simulink model "DYC_controller"  (R2018b)
settings: Solver=FixedStepAuto  StartTime=0.0  StopTime=inf  FixedStep=Ts  RelTol=1e-3  EnableMultiTasking=on
values from neighbouring files (symbols this model uses):
  A_vte = [1 0 -2*Ts*m_s/WB*(l_r*h_rc_f/w1+l_f*h_rc_r/w2) 0 -2*Ts*(K_f/w1+K_r/w2) ... (first row only)    [main.m]
  A_vte_p2 = [1 0 0 0 0 -Ts * m * hc / 2 / WB 0 -Ts * l_r * m * hc / WB / w1 ... (first row only)    [main.m]
  b1 = ones(4,1)/R    [main.m]
  boundary = 3000    [main.m]
  C_vte = [0 1 0 g 0 ... (first row only)    [main.m]
  C_vte_p2 = [1, -1, 1, -1, 0, 0, 0, 0 ... (first row only)    [main.m]
  eta = 0    [main.m]
  F_z1_s = l_r * m * g / 2 / WB    (= 9.45353456158)    [main.m]
  F_z2_s = F_z1_s    (= 9.45353456158)    [main.m]
  F_z3_s = l_f * m * g / 2 / WB    (= 9.11094809852)    [main.m]
  F_z4_s = F_z3_s    (= 9.11094809852)    [main.m]
  g = 9.81    [main.m]
  h_rc_f = 0.00    (= 0)    [main.m]
  h_rc_r = 0.00    (= 0)    [main.m]
  hc = 0.0751    [main.m]
  J = 0.9    [main.m]
  k1 = 2000    [main.m]
  k2 = 1000    [main.m]
  K_f = K_lin*l_cs^2*cos(phi*pi/180)    [main.m]
  K_r = K_lin*l_cs^2*cos(phi*pi/180)    [main.m]
  Kd = 0    [main.m]
  Ki = 75    [main.m]
  Kp = 600    [main.m]
  l_f = 0.1968    [main.m]
  l_r = 0.2042    [main.m]
  m = 3.832    [main.m]
  m_s = 0.9*m    (= 3.4488)    [main.m]
  mu = 0.8    [main.m]
  Protean_PD18_motormap = [2.92104016907 601.978033502 650.789692516 685.109940533 725.756581133 754.659963437 780.850883334 807.9513301 837.761936672 868.484372712 893.788791739 922.70944354 ... (50 elements, 25x2)]    [Protean_PD18_motormap.mat]
  Q_lat_process = 1E0*[var_r^2  0 0 0 0 0 0 0 0 ... (first row only)    [main.m]
  Q_lat_sensor = 1E-2*[var_r_s^2 0 0 0 ... (first row only)    [main.m]
  Q_meas_susp_p1 = [var_ay_m_p^2 0 0 0 ... (first row only)    [main.m]
  Q_meas_susp_p2 = [var_del_Fz^2 0 0 0 0 ... (first row only)    [main.m]
  R = 0.055    [main.m]
  Ts = 0.015    [main.m]
  V_x0 = (1000/3600)*V_x0    (= 11.1111111111)    [main.m]
  w1 = 0.2824    [main.m]
  w2 = 2.929    [main.m]
  WB = 0.406    [main.m]
undefined symbols (not defined in the file or in its folder): C_lf, C_lr, DiscIntNeverNeededParam, Discrete, t_e, Time
libraries: raspberrypilib x24, hdlsllib x21, simulink x17, discretizing x2, ctrlSharedLib x2, sharedTrackingLibrary x1
(part 1 of 3)
settings Model: SimulationMode=external  Creator=domin  LastModifiedBy=Heisenberg
settings SolverCC: ConcurrentTasks=on  PositivePriorityOrder=on  AutoInsertRateTranBlk=on
settings DataIOCC: SaveFormat=Array
settings OptimizationCC: EnhancedBackFolding=on  PassReuseOutputArgsThreshold=0  MaxStackSize=64  OptimizeBlockOrder=speed  DifferentSizesBufferReuse=on  OptimizationCustomize=off
settings DebuggingCC: ParameterTunabilityLossMsg=error  LibraryContextMissingDiagnostic=none
settings HardwareCC: ProdBitPerPointer=32  ProdBitPerSizeT=32  ProdBitPerPtrDiffT=32  ProdLargestAtomicInteger=Long  ProdLargestAtomicFloat=Double  ProdWordSize=32  ProdHWDeviceType=ARM Compatible->ARM Cortex  UseEmbeddedCoderFeatures=off  UseSimulinkCoderFeatures=off
settings ModelReferenceCC: ModelReferenceMinAlgLoopOccurrences=on
settings SFSimCC: SimUseLocalCustomCode=off  MATLABDynamicMemAlloc=off
settings RTWCC: SystemTargetFile=ert.tlc  HardwareBoard=Raspberry Pi  TLCOptions="-aInlineSetEventsForThisBaseRateFcn=TLC_FALSE -aSuppressMultiTaskScheduler=TLC_FALSE  -aRateBasedStepFcn=0"  TemplateMakefile=ert_default_tmf  RTWVerbose=off  RTWUseLocalCustomCode=off  Toolchain=GNU GCC Raspberry Pi  BuildConfiguration=Faster Runs
settings CodeAppCC: ForceParamTrailComments=on  OperatorAnnotations=on  MangleLength=10
settings ERTTargetCC: ERTCustomFileBanners=off  SupportContinuousTime=on  SupportNonInlinedSFcns=on  RemoveResetFunc=off  SupportVariableSizeSignals=on  ModelStepFunctionPrototypeControlCompliant=off  ExtMode=on  ExtModeMexArgs='192.168.1.5' 0 17725  ERTSrcFileBannerTemplate=codertarget_code_template.cgt  ERTHdrFileBannerTemplate=codertarget_code_template.cgt  ERTDataSrcFileTemplate=codertarget_code_template.cgt  ERTDataHdrFileTemplate=codertarget_code_template.cgt

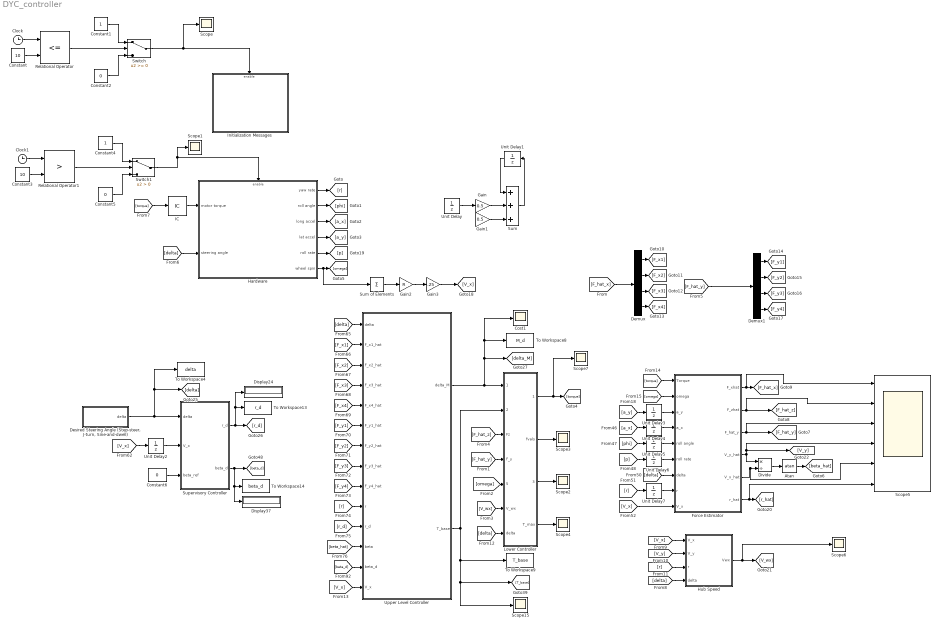
== system DYC_controller ==
  Atan : Trigonometry  Operator=atan
  Clock : Clock
  Clock1 : Clock
  Constant : Constant  Value=10
  Constant1 : Constant
  Constant2 : Constant  Value=0
  Constant3 : Constant  Value=10
  Constant4 : Constant
  Constant5 : Constant  Value=0
  Constant6 : Constant  Value=0  SampleTime=Ts
  Cost1 : Scope
  Demux : Demux
  Demux1 : Demux
  "Desired Steering Angle (Step-steer, J-turn, Sine-and-dwell)" : Subsystem
  Display24 : Display
  Display37 : Display
  Divide : Product  Inputs=*/
  Force Estimator : Subsystem
  Gain : Gain  Gain=0.5
  Gain1 : Gain  Gain=0.5
  Gain2 : Gain  Gain=R
  Gain3 : Gain  Gain=.25
  Hardware : Subsystem
  Hub Speed : Subsystem
  IC : InitialCondition  Value=0
  Initialization Messages : Subsystem
  Lower Controller : Subsystem
  Relational Operator : RelationalOperator  Operator=<=  OutDataTypeStr=boolean  RndMeth=Simplest
  Relational Operator1 : RelationalOperator  Operator=>  OutDataTypeStr=boolean  RndMeth=Simplest
  Scope{,1..4,6..7,15} (8 alike) : Scope
  Scope5 : Scope  NumInputPorts=6
  Sum : Sum  Inputs=+++
  Sum of Elements : Sum  Inputs=+
  "Supervisory Controller " : Subsystem
  Switch : Switch
  Switch1 : Switch  Criteria=u2 > Threshold
  To Workspace13 : ToWorkspace  VariableName=r_d  SampleTime=-1
  To Workspace14 : ToWorkspace  VariableName=beta_d  SampleTime=-1
  To Workspace4 : ToWorkspace  VariableName=delta  SampleTime=-1
  To Workspace8 : ToWorkspace  VariableName=M_d  SampleTime=-1
  To Workspace9 : ToWorkspace  VariableName=T_base  SampleTime=-1
  Unit Delay{,1..7} (8 alike) : UnitDelay  SampleTime=-1
  Upper Level Controller : Subsystem
  wires:
  Clock/1 -> Relational Operator/1
  Constant/1 -> Relational Operator/2
  Relational Operator/1 -> Switch/2
  Constant1/1 -> Switch/1
  Constant2/1 -> Switch/3
  Switch/1 -> Scope/1, Initialization Messages/Enable
  Switch1/1 -> Scope1/1, Hardware/Enable
  Constant5/1 -> Switch1/3
  Constant4/1 -> Switch1/1
  Relational Operator1/1 -> Switch1/2
  Constant3/1 -> Relational Operator1/2
  Clock1/1 -> Relational Operator1/1
  "Supervisory Controller "/1(r_d) -> Display24/1, To Workspace13/1, [r_d]
  Constant6/1 -> "Supervisory Controller "/3(beta_ref)
  [V_x] -> Unit Delay2/1
  "Desired Steering Angle (Step-steer, J-turn, Sine-and-dwell)"/1(delta) -> To Workspace4/1, [delta], "Supervisory Controller "/1(delta)
  "Supervisory Controller "/2(beta_d) -> To Workspace14/1, Display37/1, [beta_d]
  [F_x1] -> Upper Level Controller/2(F_x1_hat)
  [delta] -> Lower Controller/7(delta)
  [F_y3] -> Upper Level Controller/8(F_y3_hat)
  Upper Level Controller/1(delta_M) -> Cost1/1, To Workspace8/1, [delta_M], Lower Controller/1(delta_M)
  [F_x3] -> Upper Level Controller/4(F_x3_hat)
  [F_y1] -> Upper Level Controller/6(F_y1_hat)
  [F_y4] -> Upper Level Controller/9(F_y4_hat)
  Upper Level Controller/2(T_base) -> To Workspace9/1, [T_base], Scope15/1, Lower Controller/2(T_base)
  [F_hat_y] -> Lower Controller/4(F_y)
  [r_d] -> Upper Level Controller/11(r_d)
  [F_x4] -> Upper Level Controller/5(F_x4_hat)
  [V_wx] -> Lower Controller/6(V_wx)
  [r] -> Upper Level Controller/10(r)
  [V_x] -> Upper Level Controller/14(V_x)
  [delta] -> Upper Level Controller/1(delta)
  [beta_d] -> Upper Level Controller/13(beta_d)
  [F_hat_z] -> Lower Controller/3(Fz)
  [F_x2] -> Upper Level Controller/3(F_x2_hat)
  [omega] -> Lower Controller/5(omega)
  [F_y2] -> Upper Level Controller/7(F_y2_hat)
  [beta_hat] -> Upper Level Controller/12(beta)
  [torque] -> Force Estimator/1(Torque)
  [a_y] -> Unit Delay3/1
  [p] -> Unit Delay6/1
  [delta] -> Force Estimator/7(delta)
  [a_x] -> Unit Delay4/1
  [r] -> Unit Delay7/1
  [phi] -> Unit Delay5/1
  [omega] -> Force Estimator/2(omega)
  Hardware/1(yaw rate) -> [r]
  Hardware/2(roll angle) -> [phi]
  Hardware/3(long accel) -> [a_x]
  Hardware/4(lat accel) -> [a_y]
  Hardware/6(wheel spin) -> Sum of Elements/1, [omega]
  Divide/1 -> Atan/1
  Force Estimator/4(V_y_hat) -> Scope5/4, [V_y], Divide/1
  Force Estimator/5(V_x_hat) -> Scope5/5, Divide/2
  Atan/1 -> [beta_hat]
  Force Estimator/3(F_hat_y) -> Scope5/3, [F_hat_y]
  Force Estimator/2(F_zhat) -> Scope5/2, [F_hat_z]
  Force Estimator/1(F_xhat) -> Scope5/1, [F_hat_x]
  [F_hat_x] -> Demux/1
  Demux/1 -> [F_x1]
  Demux/2 -> [F_x2]
  Demux/3 -> [F_x3]
  Demux/4 -> [F_x4]
  Demux1/4 -> [F_y4]
  Demux1/3 -> [F_y3]
  Demux1/2 -> [F_y2]
  Demux1/1 -> [F_y1]
  Unit Delay/1 -> Gain/1
  Gain/1 -> Sum/2
  Gain1/1 -> Sum/3
  Hardware/5(roll rate) -> [p]
  [delta] -> Hardware/2(steering angle)
  Force Estimator/6(r_hat) -> Scope5/6, [r_hat]
  Lower Controller/3(iterations) -> Scope2/1
  Lower Controller/2(fvals) -> Scope3/1
  Lower Controller/4(T_max) -> Scope4/1
  [delta] -> Hub Speed/4(delta)
  [V_y] -> Hub Speed/2(V_y)
  [r] -> Hub Speed/3(r)
  [V_x] -> Hub Speed/1("V_x ")
  Hub Speed/1(Vwx) -> Scope6/1, [V_wx]
  Lower Controller/1(Motor Torques) -> Scope7/1, [torque]
  [torque] -> IC/1
  [F_hat_y] -> Demux1/1
  Unit Delay1/1 -> Sum/1
  Unit Delay2/1 -> "Supervisory Controller "/2(V_x)
  IC/1 -> Hardware/1(motor torque)
  Unit Delay3/1 -> Force Estimator/3(a_y)
  Unit Delay4/1 -> Force Estimator/4(a_x)
  Unit Delay5/1 -> Force Estimator/5(roll angle)
  Unit Delay6/1 -> Force Estimator/6(roll rate)
  Unit Delay7/1 -> Force Estimator/8(r)
  [V_x] -> Force Estimator/9(V_x)
  Sum/1 -> Unit Delay1/1
  Sum of Elements/1 -> Gain2/1
  Gain2/1 -> Gain3/1
  Gain3/1 -> [V_x]

== system DYC_controller/Desired Steering Angle (Step-steer, J-turn, Sine-and-dwell) ==
  J-Turn : Subsystem
  delta : Outport
  wires:
  J-Turn/1(delta) -> delta/1

== system DYC_controller/Force Estimator ==
  Torque : Inport
  omega : Inport  Port=2
  a_y : Inport  Port=3
  a_x : Inport  Port=4
  roll angle : Inport  Port=5
  roll rate : Inport  Port=6
  delta : Inport  Port=7
  r : Inport  Port=8
  V_x : Inport  Port=9
  Gain : Gain  Gain=pi/180
  Gain1 : Gain  Gain=pi/180
  Gain2 : Gain  Gain=pi/180
  Lateral Tire Force Estimation : Subsystem
  Longitudinal Tire Force Estimation : Subsystem
  Mux : Mux
  Vertical Tire Force Estimation : Subsystem
  F_xhat : Outport
  F_zhat : Outport  Port=2
  F_hat_y : Outport  Port=3
  V_y_hat : Outport  Port=4
  V_x_hat : Outport  Port=5
  r_hat : Outport  Port=6
  wires:
  Torque/1 -> Longitudinal Tire Force Estimation/1(torque)
  Longitudinal Tire Force Estimation/1(F_hat_x1) -> Mux/1
  Longitudinal Tire Force Estimation/2(F_hat_x2) -> Mux/2
  Longitudinal Tire Force Estimation/3(F_hat_x3) -> Mux/3
  Longitudinal Tire Force Estimation/4(F_hat_x4) -> Mux/4
  Mux/1 -> F_xhat/1
  omega/1 -> Longitudinal Tire Force Estimation/2(omega)
  a_y/1 -> Vertical Tire Force Estimation/4(a_y)
  a_x/1 -> Vertical Tire Force Estimation/1(a_x)
  roll angle/1 -> Gain/1
  roll rate/1 -> Gain1/1
  delta/1 -> Lateral Tire Force Estimation/2(delta)
  r/1 -> Gain2/1
  V_x/1 -> Lateral Tire Force Estimation/4(V_x)
  Lateral Tire Force Estimation/1(r_hat) -> r_hat/1
  Vertical Tire Force Estimation/2(a_x_hat) -> Lateral Tire Force Estimation/5(a_x)
  Vertical Tire Force Estimation/3(a_y_hat) -> Lateral Tire Force Estimation/6(a_y)
  Vertical Tire Force Estimation/1(F_zhat) -> F_zhat/1, Lateral Tire Force Estimation/1(F_zhat)
  Lateral Tire Force Estimation/4(F_hat_y) -> F_hat_y/1
  Lateral Tire Force Estimation/3(V_y_hat) -> V_y_hat/1
  Lateral Tire Force Estimation/2(V_x_hat) -> V_x_hat/1
  Gain/1 -> Vertical Tire Force Estimation/2(roll angle)
  Gain1/1 -> Vertical Tire Force Estimation/3(roll rate)
  Gain2/1 -> Lateral Tire Force Estimation/3(r)

== system DYC_controller/Hardware ==
  motor torque : Inport
  steering angle : Inport  Port=2
  Enable : EnablePort
  Const Mot Vel : Constant  Value=50
  SSIV Hardware Communication : Subsystem
  Throttle and Steering Handler : Subsystem
  yaw rate : Outport
  roll angle : Outport  Port=2
  long accel : Outport  Port=3
  lat accel : Outport  Port=4
  roll rate : Outport  Port=5
  wheel spin : Outport  Port=6
  wires:
  Throttle and Steering Handler/1(Throttle RF) -> SSIV Hardware Communication/1(throttle_right_front)
  Throttle and Steering Handler/2(Throttle LF) -> SSIV Hardware Communication/2(throttle_left_front)
  Throttle and Steering Handler/3(Throttle RR) -> SSIV Hardware Communication/3(throttle_right_rear)
  Throttle and Steering Handler/4(Throttle LR) -> SSIV Hardware Communication/4(throttle_left_rear)
  Throttle and Steering Handler/5(Outport) -> SSIV Hardware Communication/5(servo_out)
  Const Mot Vel/1 -> Throttle and Steering Handler/2(Inport2)
  SSIV Hardware Communication/9(gyr_z) -> yaw rate/1
  SSIV Hardware Communication/3(euler_roll) -> roll angle/1
  SSIV Hardware Communication/4(acc_x) -> long accel/1
  SSIV Hardware Communication/6(acc_y) -> lat accel/1
  motor torque/1 -> Throttle and Steering Handler/1(throttle)
  steering angle/1 -> Throttle and Steering Handler/3(steering angle)
  SSIV Hardware Communication/7(gyr_y) -> roll rate/1
  SSIV Hardware Communication/12(wheel spin) -> wheel spin/1

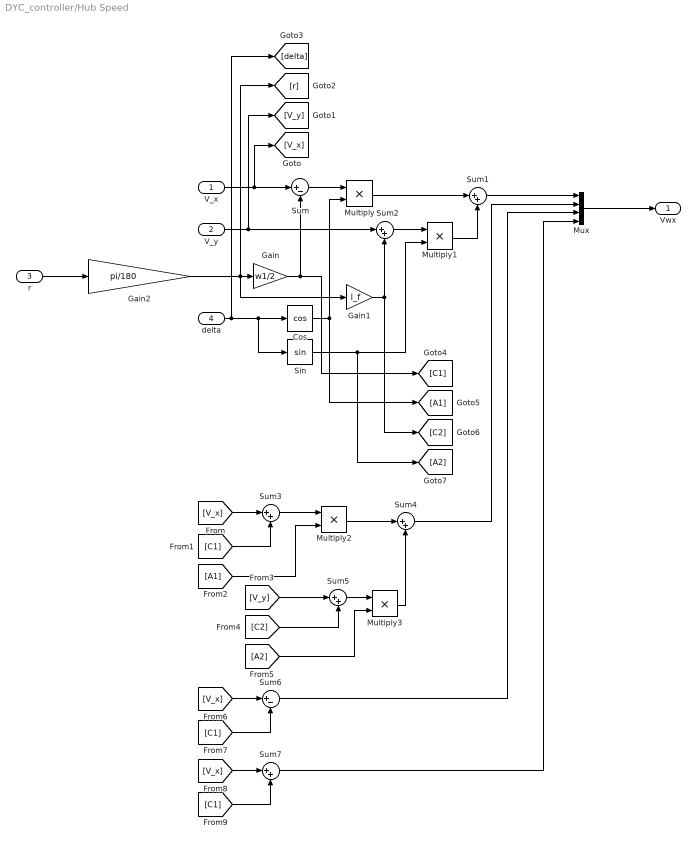
== system DYC_controller/Hub Speed ==
  "V_x " : Inport
  V_y : Inport  Port=2
  r : Inport  Port=3
  delta : Inport  Port=4
  Cos : Trigonometry  Operator=cos
  Gain : Gain  Gain=w1/2
  Gain1 : Gain  Gain=l_f
  Gain2 : Gain  Gain=pi/180
  Multiply{,1..3} (4 alike) : Product
  Mux : Mux
  Sin : Trigonometry
  Sum : Sum  Inputs=|+-
  Sum{1..5,7} (6 alike) : Sum  Inputs=|++
  Sum6 : Sum  Inputs=|+-
  Vwx : Outport
  wires:
  r/1 -> Gain2/1
  Gain/1 -> Sum/2, [C1]
  Sum/1 -> Multiply/1
  Cos/1 -> [A1], Multiply/2
  Multiply/1 -> Sum1/1
  V_y/1 -> [V_y], Sum2/1
  Gain1/1 -> [C2], Sum2/2
  Sum2/1 -> Multiply1/1
  Sin/1 -> [A2], Multiply1/2
  Multiply1/1 -> Sum1/2
  Sum1/1 -> Mux/1
  Mux/1 -> Vwx/1
  "V_x "/1 -> [V_x], Sum/1
  delta/1 -> [delta], Sin/1, Cos/1
  [V_x] -> Sum3/1
  [C1] -> Sum3/2
  Sum3/1 -> Multiply2/1
  [A1] -> Multiply2/2
  Multiply2/1 -> Sum4/1
  Sum5/1 -> Multiply3/1
  Multiply3/1 -> Sum4/2
  [V_y] -> Sum5/1
  [C2] -> Sum5/2
  [A2] -> Multiply3/2
  Sum4/1 -> Mux/2
  [C1] -> Sum6/2
  Sum6/1 -> Mux/3
  [V_x] -> Sum6/1
  [V_x] -> Sum7/1
  Sum7/1 -> Mux/4
  [C1] -> Sum7/2
  Gain2/1 -> [r], Gain1/1, Gain/1

== system DYC_controller/Initialization Messages ==
  Enable : EnablePort
  Dead Switch : Constant  OutDataTypeStr=uint8
  Display{1..8} (8 alike) : Display
      settings: Format=decimal (Stored Integer)
  IMU Reset : Constant  OutDataTypeStr=uint8
  Motor Controllers On : Constant  OutDataTypeStr=uint8
  Print the imu data on the Teensy : Constant  Value=0  OutDataTypeStr=uint8
  Print the radio tranceiver data on the Teensy : Constant  Value=0  OutDataTypeStr=uint8
  Print the register map on the Teensy : Constant  Value=0  OutDataTypeStr=uint8
  SPI Register Write begin_data_collection : raspberrypilib/SPI Register Write  BoardProperty=Pi 3 Model B  SPIModule=uint32(0)  Mode=Master  BusSpeed=1000000  Pin=SPI0_CE1  FirstBitToTransfer=Most significant bit (MSB)  ClockMode=0  BlockFunction=Write  RegisterAddress=1  OutputDataType=int8  OutputDataLength=1
      settings: SourceProductName=Simulink Support Package for Raspberry Pi Hardware  SourceProductBaseCode=RASPPI
  SPI Register Write dead_switch : raspberrypilib/SPI Register Write  BoardProperty=Pi 3 Model B  SPIModule=uint32(0)  Mode=Master  BusSpeed=1000000  Pin=SPI0_CE1  FirstBitToTransfer=Most significant bit (MSB)  ClockMode=0  BlockFunction=Write  RegisterAddress=7  OutputDataType=int8  OutputDataLength=1
      settings: SourceProductName=Simulink Support Package for Raspberry Pi Hardware  SourceProductBaseCode=RASPPI
  SPI Register Write init_motor_controllers : raspberrypilib/SPI Register Write  BoardProperty=Pi 3 Model B  SPIModule=uint32(0)  Mode=Master  BusSpeed=1000000  Pin=SPI0_CE1  FirstBitToTransfer=Most significant bit (MSB)  ClockMode=0  BlockFunction=Write  RegisterAddress=5  OutputDataType=int8  OutputDataLength=1
      settings: SourceProductName=Simulink Support Package for Raspberry Pi Hardware  SourceProductBaseCode=RASPPI
  SPI Register Write init_servo_radio : raspberrypilib/SPI Register Write  BoardProperty=Pi 3 Model B  SPIModule=uint32(0)  Mode=Master  BusSpeed=1000000  Pin=SPI0_CE1  FirstBitToTransfer=Most significant bit (MSB)  ClockMode=0  BlockFunction=Write  RegisterAddress=4  OutputDataType=int8  OutputDataLength=1
      settings: SourceProductName=Simulink Support Package for Raspberry Pi Hardware  SourceProductBaseCode=RASPPI
  SPI Register Write print_imu ENSURING NO PRINTING OCCURS DURING DYNAMIC OP UNLESS EXPLICITLY SET : raspberrypilib/SPI Register Write  BoardProperty=Pi 3 Model B  SPIModule=uint32(0)  Mode=Master  BusSpeed=1000000  Pin=SPI0_CE1  FirstBitToTransfer=Most significant bit (MSB)  ClockMode=0  BlockFunction=Write  RegisterAddress=2  OutputDataType=int8  OutputDataLength=1
      settings: SourceProductName=Simulink Support Package for Raspberry Pi Hardware  SourceProductBaseCode=RASPPI
  SPI Register Write print_radio ENSURING NO PRINTING OCCURS DURING DYNAMIC OP UNLESS EXPLICITLY SET : raspberrypilib/SPI Register Write  BoardProperty=Pi 3 Model B  SPIModule=uint32(0)  Mode=Master  BusSpeed=1000000  Pin=SPI0_CE1  FirstBitToTransfer=Most significant bit (MSB)  ClockMode=0  BlockFunction=Write  RegisterAddress=3  OutputDataType=int8  OutputDataLength=1
      settings: SourceProductName=Simulink Support Package for Raspberry Pi Hardware  SourceProductBaseCode=RASPPI
  SPI Register Write print_registers ENSURING NO PRINTING OCCURS DURING DYNAMIC OP UNLESS EXPLICITLY SET : raspberrypilib/SPI Register Write  BoardProperty=Pi 3 Model B  SPIModule=uint32(0)  Mode=Master  BusSpeed=1000000  Pin=SPI0_CE1  FirstBitToTransfer=Most significant bit (MSB)  ClockMode=0  BlockFunction=Write  RegisterAddress=0  OutputDataType=int8  OutputDataLength=1
      settings: SourceProductName=Simulink Support Package for Raspberry Pi Hardware  SourceProductBaseCode=RASPPI
  SPI Register Write reset_imu : raspberrypilib/SPI Register Write  BoardProperty=Pi 3 Model B  SPIModule=uint32(0)  Mode=Master  BusSpeed=1000000  Pin=SPI0_CE1  FirstBitToTransfer=Most significant bit (MSB)  ClockMode=0  BlockFunction=Write  RegisterAddress=6  OutputDataType=int8  OutputDataLength=1
      settings: SourceProductName=Simulink Support Package for Raspberry Pi Hardware  SourceProductBaseCode=RASPPI
  Servo and Radio On : Constant  OutDataTypeStr=uint8
  Take Data : Constant  OutDataTypeStr=uint8
  wires:
  Take Data/1 -> Display1/1, SPI Register Write begin_data_collection/1
  Servo and Radio On/1 -> SPI Register Write init_servo_radio/1, Display2/1
  Motor Controllers On/1 -> Display3/1, SPI Register Write init_motor_controllers/1
  IMU Reset/1 -> SPI Register Write reset_imu/1, Display4/1
  Dead Switch/1 -> Display5/1, SPI Register Write dead_switch/1
  Print the register map on the Teensy/1 -> SPI Register Write print_registers ENSURING NO PRINTING OCCURS DURING DYNAMIC OP UNLESS EXPLICITLY SET/1, Display6/1
  Print the imu data on the Teensy/1 -> SPI Register Write print_imu ENSURING NO PRINTING OCCURS DURING DYNAMIC OP UNLESS EXPLICITLY SET/1, Display7/1
  Print the radio tranceiver data on the Teensy/1 -> Display8/1, SPI Register Write print_radio ENSURING NO PRINTING OCCURS DURING DYNAMIC OP UNLESS EXPLICITLY SET/1

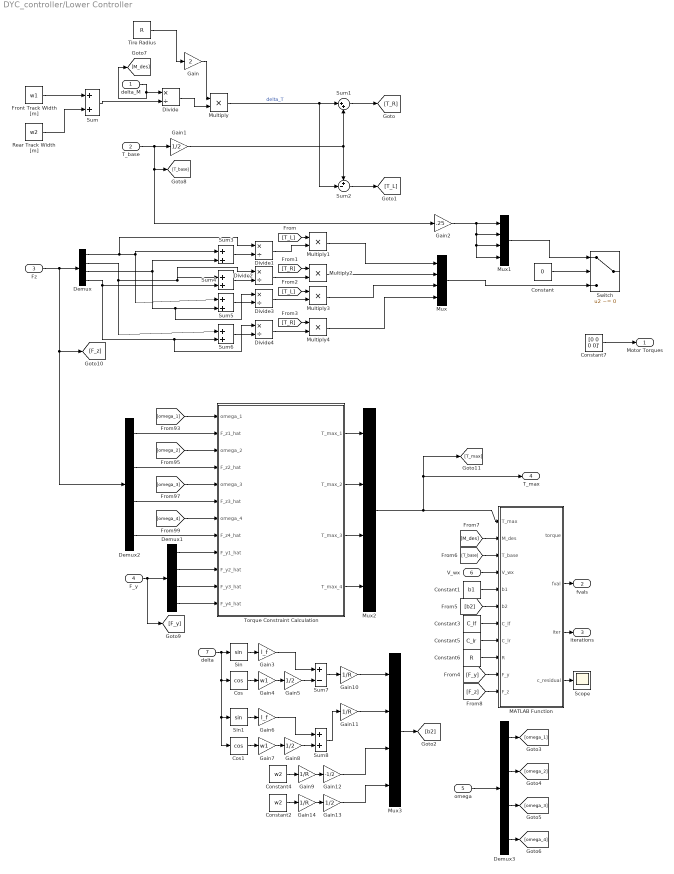
== system DYC_controller/Lower Controller ==
  delta_M : Inport
  T_base : Inport  Port=2
  Fz : Inport  Port=3
  F_y : Inport  Port=4
  omega : Inport  Port=5
  V_wx : Inport  Port=6
  delta : Inport  Port=7
  Constant : Constant  Value=0
  Constant1 : Constant  Value=b1
  Constant2 : Constant  Value=w2
  Constant3 : Constant  Value=C_lf
  Constant4 : Constant  Value=w2
  Constant5 : Constant  Value=C_lr
  Constant6 : Constant  Value=R
  Constant7 : Constant  Value=[0 0 0 0]'
  Cos : Trigonometry  Operator=cos
  Cos1 : Trigonometry  Operator=cos
  Demux{,1..3} (4 alike) : Demux
  Divide{,1..4} (5 alike) : Product  Inputs=*/
  Front Track Width [m] : Constant  Value=w1
  Gain : Gain  Gain=2
  Gain{1,5,8,13} (4 alike) : Gain  Gain=1/2
  Gain{9..11,14} (4 alike) : Gain  Gain=1/R
  Gain12 : Gain  Gain=-1/2
  Gain2 : Gain  Gain=.25
  Gain3 : Gain  Gain=l_f
  Gain4 : Gain  Gain=w1
  Gain6 : Gain  Gain=l_f
  Gain7 : Gain  Gain=w1
  MATLAB Function : MATLAB Function  TreatAsAtomicUnit=on
  Multiply{,1..4} (5 alike) : Product
  Mux{,1..3} (4 alike) : Mux
  Rear Track Width [m] : Constant  Value=w2
  Scope : Scope
  Sin : Trigonometry
  Sin1 : Trigonometry
  Sum : Sum
  Sum{1,3..6} (5 alike) : Sum  Inputs=|++
  Sum2 : Sum  Inputs=+-|
  Sum7 : Sum  Inputs=+-
  Sum8 : Sum
  Switch : Switch  Criteria=u2 ~= 0
  Tire Radius : Constant  Value=R
  Torque Constraint Calculation : Subsystem
  Motor Torques : Outport
  fvals : Outport  Port=2
  iterations : Outport  Port=3
  T_max : Outport  Port=4
  wires:
  Front Track Width [m]/1 -> Sum/1
  Rear Track Width [m]/1 -> Sum/2
  Sum/1 -> Divide/2
  delta_M/1 -> [M_des], Divide/1
  Divide/1 -> Multiply/2
  Tire Radius/1 -> Gain/1
  Gain/1 -> Multiply/1
  Multiply/1 -> Sum2/2, Sum1/1  "delta_T"
  Sum1/1 -> [T_R]
  Sum2/1 -> [T_L]
  Demux/1 -> Sum5/1, Sum3/1, Divide1/1
  Demux/3 -> Divide3/1, Sum5/2, Sum3/2
  Sum3/1 -> Divide1/2
  Divide1/1 -> Multiply1/2
  [T_L] -> Multiply1/1
  Demux/2 -> Sum6/1, Divide2/1, Sum4/1
  Demux/4 -> Divide4/1, Sum6/2, Sum4/2
  Sum4/1 -> Divide2/2
  Divide2/1 -> Multiply2/2
  [T_R] -> Multiply2/1
  Sum5/1 -> Divide3/2
  Divide3/1 -> Multiply3/2
  [T_L] -> Multiply3/1
  Sum6/1 -> Divide4/2
  Divide4/1 -> Multiply4/2
  [T_R] -> Multiply4/1
  T_base/1 -> [T_base], Gain2/1, Gain1/1
  Gain1/1 -> Sum2/1, Sum1/2
  Multiply1/1 -> Mux/1
  Multiply2/1 -> Mux/2
  Multiply3/1 -> Mux/3
  Multiply4/1 -> Mux/4
  Mux/1 -> Switch/3
  Gain2/1 -> Mux1/4, Mux1/3, Mux1/2, Mux1/1
  Mux1/1 -> Switch/1
  Constant/1 -> Switch/2
  Demux2/3 -> Torque Constraint Calculation/6(F_z3_hat)
  Demux2/2 -> Torque Constraint Calculation/4(F_z2_hat)
  [omega_4] -> Torque Constraint Calculation/7(omega_4)
  Demux2/1 -> Torque Constraint Calculation/2(F_z1_hat)
  [omega_1] -> Torque Constraint Calculation/1(omega_1)
  Demux2/4 -> Torque Constraint Calculation/8(F_z4_hat)
  [omega_3] -> Torque Constraint Calculation/5(omega_3)
  [omega_2] -> Torque Constraint Calculation/3(omega_2)
  Torque Constraint Calculation/1(T_max_1) -> Mux2/1
  Torque Constraint Calculation/2(T_max_2) -> Mux2/2
  Torque Constraint Calculation/3(T_max_3) -> Mux2/3
  Torque Constraint Calculation/4(T_max_4) -> Mux2/4
  Demux1/1 -> Torque Constraint Calculation/9(F_y1_hat)
  Demux1/2 -> Torque Constraint Calculation/10(F_y2_hat)
  Demux1/3 -> Torque Constraint Calculation/11(F_y3_hat)
  Demux1/4 -> Torque Constraint Calculation/12(F_y4_hat)
  F_y/1 -> [F_y], Demux1/1
  Mux2/1 -> [T_max], T_max/1, MATLAB Function/1(T_max)
  Constant1/1 -> MATLAB Function/5(b1)
  Sin/1 -> Gain3/1
  Cos/1 -> Gain4/1
  Gain4/1 -> Gain5/1
  Gain5/1 -> Sum7/2
  Gain3/1 -> Sum7/1
  Sum7/1 -> Gain10/1
  Gain7/1 -> Gain8/1
  delta/1 -> Cos1/1, Sin1/1, Cos/1, Sin/1
  Gain6/1 -> Sum8/1
  Gain8/1 -> Sum8/2
  Cos1/1 -> Gain7/1
  Sum8/1 -> Gain11/1
  Sin1/1 -> Gain6/1
  Constant4/1 -> Gain9/1
  Gain9/1 -> Gain12/1
  Gain14/1 -> Gain13/1
  Constant2/1 -> Gain14/1
  Gain10/1 -> Mux3/1
  Gain11/1 -> Mux3/2
  Gain12/1 -> Mux3/3
  Gain13/1 -> Mux3/4
  Mux3/1 -> [b2]
  [b2] -> MATLAB Function/6(b2)
  Constant3/1 -> MATLAB Function/7(C_lf)
  Constant5/1 -> MATLAB Function/8(C_lr)
  omega/1 -> Demux3/1
  Demux3/1 -> [omega_1]
  Demux3/2 -> [omega_2]
  Demux3/3 -> [omega_3]
  Demux3/4 -> [omega_4]
  V_wx/1 -> MATLAB Function/4(V_wx)
  [T_base] -> MATLAB Function/3(T_base)
  [M_des] -> MATLAB Function/2(M_des)
  MATLAB Function/2(fval) -> fvals/1
  MATLAB Function/3(iter) -> iterations/1
  MATLAB Function/4(c_residual) -> Scope/1
  Constant6/1 -> MATLAB Function/9(R)
  Fz/1 -> [F_z], Demux2/1, Demux/1
  [F_y] -> MATLAB Function/10(F_y)
  [F_z] -> MATLAB Function/11(F_z)
  Constant7/1 -> Motor Torques/1

== system DYC_controller/Supervisory Controller  ==
  delta : Inport
  V_x : Inport  Port=2
  beta_ref : Inport  Port=3
  Atan : Trigonometry  Operator=atan
  Constant : Constant  Value=WB
  Constant1 : Constant
  Constant5 : Constant  Value=.02
  "Desired Understeer Gradient (US: K>0, NS: K=0, OS: K<0)" : Constant  Value=0
  Divide : Product  Inputs=*/
  Divide2 : Product  Inputs=*/
  Gain : Gain  Gain=mu
  Gain1 : Gain  Gain=g
  Gain10 : Gain  Gain=g
  Gain7 : Gain  Gain=-1
  Gain8 : Gain  Gain=-1
  Gain9 : Gain  Gain=mu
  Multiply : Product
  Saturation Dynamic : simulink/Discontinuities/Saturation Dynamic  OutMin=[]  OutMax=[]  OutDataTypeStr=Inherit: Same as second input  OutDataType=fixdt(1, 16)  OutScaling=2^-10  DoSatur=off
  Saturation Dynamic1 : simulink/Discontinuities/Saturation Dynamic  OutMin=[]  OutMax=[]  OutDataTypeStr=Inherit: Same as second input  OutDataType=fixdt(1, 16)  OutScaling=2^-10  DoSatur=off
  Scope : Scope  NumInputPorts=3
  Sum : Sum
  r_d : Outport
  beta_d : Outport  Port=2
  wires:
  delta/1 -> Multiply/1
  V_x/1 -> Multiply/2, Divide2/2
  Multiply/1 -> Divide/1
  Constant/1 -> Sum/1
  Sum/1 -> Divide/2
  Saturation Dynamic/1 -> r_d/1
  Divide2/1 -> Gain7/1, Saturation Dynamic/1, Scope/1
  Gain7/1 -> Scope/3, Saturation Dynamic/3
  Divide/1 -> Scope/2, Saturation Dynamic/2
  Constant5/1 -> Gain9/1
  Gain9/1 -> Gain10/1
  Gain10/1 -> Atan/1
  Atan/1 -> Gain8/1, Saturation Dynamic1/1
  Gain8/1 -> Saturation Dynamic1/3
  beta_ref/1 -> Saturation Dynamic1/2
  Saturation Dynamic1/1 -> beta_d/1
  "Desired Understeer Gradient (US: K>0, NS: K=0, OS: K<0)"/1 -> Sum/2
  Constant1/1 -> Gain1/1
  Gain/1 -> Divide2/1
  Gain1/1 -> Gain/1

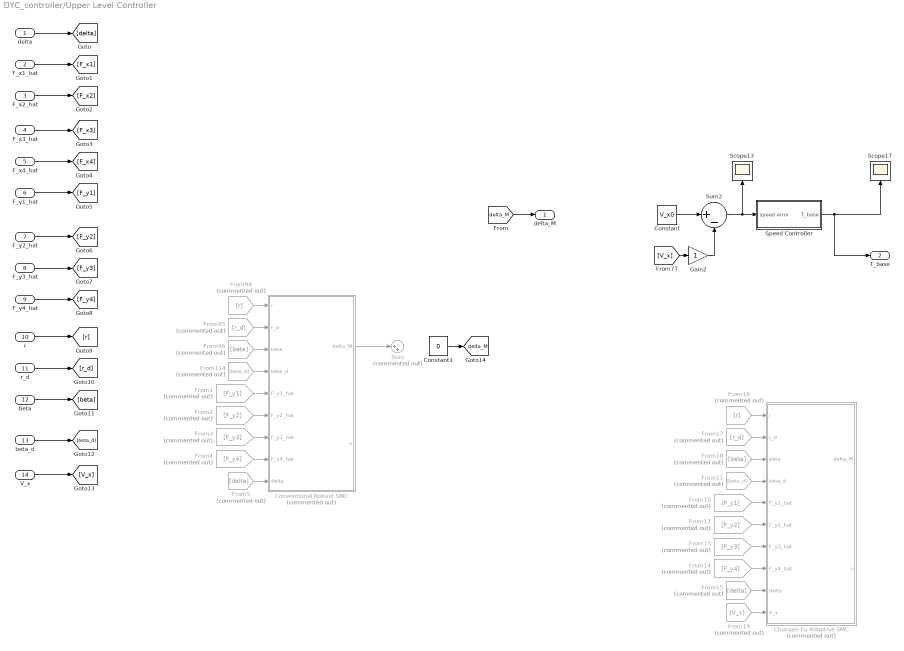
== system DYC_controller/Upper Level Controller ==
  delta : Inport
  F_x1_hat : Inport  Port=2
  F_x2_hat : Inport  Port=3
  F_x3_hat : Inport  Port=4
  F_x4_hat : Inport  Port=5
  F_y1_hat : Inport  Port=6
  F_y2_hat : Inport  Port=7
  F_y3_hat : Inport  Port=8
  F_y4_hat : Inport  Port=9
  r : Inport  Port=10
  r_d : Inport  Port=11
  beta : Inport  Port=12
  beta_d : Inport  Port=13
  V_x : Inport  Port=14
  Chunyen Fu Adaptive SMC : Subsystem  Commented=on
  Constant : Constant  Value=V_x0
  Constant1 : Constant  Value=0  SampleTime=Ts
  Conventional Robust SMC : Subsystem  Commented=on
  From1 : From  Commented=on  GotoTag=F_y1
  From10 : From  Commented=on  GotoTag=F_y1
  From11 : From  Commented=on  GotoTag=beta_d
  From114 : From  Commented=on  GotoTag=beta_d
  From12 : From  Commented=on  GotoTag=F_y2
  From13 : From  Commented=on  GotoTag=F_y3
  From14 : From  Commented=on  GotoTag=F_y4
  From15 : From  Commented=on  GotoTag=delta
  From16 : From  Commented=on  GotoTag=r
  From17 : From  Commented=on  GotoTag=r_d
  From18 : From  Commented=on  GotoTag=beta
  From19 : From  Commented=on  GotoTag=V_x
  From2 : From  Commented=on  GotoTag=F_y2
  From3 : From  Commented=on  GotoTag=F_y3
  From4 : From  Commented=on  GotoTag=F_y4
  From5 : From  Commented=on  GotoTag=delta
  From94 : From  Commented=on  GotoTag=r
  From95 : From  Commented=on  GotoTag=r_d
  From96 : From  Commented=on  GotoTag=beta
  Gain2 : Gain
  Scope13 : Scope
  Scope17 : Scope
  Speed Controller : Subsystem
  Sum : Sum  Commented=on  Inputs=|++
  Sum2 : Sum  Inputs=|+-
  delta_M : Outport
  T_base : Outport  Port=2
  tag scope: delta_M=global
  wires:
  delta/1 -> [delta]
  F_x1_hat/1 -> [F_x1]
  F_x2_hat/1 -> [F_x2]
  F_x3_hat/1 -> [F_x3]
  F_y1_hat/1 -> [F_y1]
  F_x4_hat/1 -> [F_x4]
  F_y2_hat/1 -> [F_y2]
  F_y4_hat/1 -> [F_y4]
  F_y3_hat/1 -> [F_y3]
  r/1 -> [r]
  beta/1 -> [beta]
  r_d/1 -> [r_d]
  beta_d/1 -> [beta_d]
  From96/1 -> Conventional Robust SMC/3(beta)
  From114/1 -> Conventional Robust SMC/4(beta_d)
  From95/1 -> Conventional Robust SMC/2(r_d)
  From94/1 -> Conventional Robust SMC/1(r)
  [delta_M] -> delta_M/1
  Gain2/1 -> Sum2/2
  Constant/1 -> Sum2/1
  [V_x] -> Gain2/1
  Sum2/1 -> Speed Controller/1(speed error), Scope13/1
  V_x/1 -> [V_x]
  Speed Controller/1(T_base) -> Scope17/1, T_base/1
  From1/1 -> Conventional Robust SMC/5(F_y1_hat)
  From2/1 -> Conventional Robust SMC/6(F_y2_hat)
  From3/1 -> Conventional Robust SMC/7(F_y3_hat)
  From4/1 -> Conventional Robust SMC/8(F_y4_hat)
  From5/1 -> Conventional Robust SMC/9(delta)
  Conventional Robust SMC/1(delta_M) -> Sum/1
  From16/1 -> Chunyen Fu Adaptive SMC/1(r)
  From11/1 -> Chunyen Fu Adaptive SMC/4(beta_d)
  From15/1 -> Chunyen Fu Adaptive SMC/9(delta)
  From13/1 -> Chunyen Fu Adaptive SMC/7(F_y3_hat)
  From14/1 -> Chunyen Fu Adaptive SMC/8(F_y4_hat)
  From18/1 -> Chunyen Fu Adaptive SMC/3(beta)
  From10/1 -> Chunyen Fu Adaptive SMC/5(F_y1_hat)
  From12/1 -> Chunyen Fu Adaptive SMC/6(F_y2_hat)
  From17/1 -> Chunyen Fu Adaptive SMC/2(r_d)
  From19/1 -> Chunyen Fu Adaptive SMC/10(V_x)
  Constant1/1 -> [delta_M]

== system DYC_controller/Desired Steering Angle (Step-steer, J-turn, Sine-and-dwell)/J-Turn ==
  Constant : Constant  Value=10
  Gain5 : Gain  Gain=pi/180
  Ramp : discretizing/Discretized Ramp  slope=10  start=10  X0=0  SampleTime=Ts
  Ramp1 : discretizing/Discretized Ramp  slope=-10  start=11  X0=0  SampleTime=Ts
  Scope12 : Scope
  Scope22 : Scope
  Sum3 : Sum  Inputs=|++
  delta : Outport
  wires:
  Sum3/1 -> Gain5/1, Scope12/1
  Gain5/1 -> Scope22/1, delta/1  "[rad]"
  Constant/1 -> Sum3/1

== system DYC_controller/Force Estimator/Lateral Tire Force Estimation ==
  F_zhat : Inport
  delta : Inport  Port=2
  r : Inport  Port=3
  V_x : Inport  Port=4
  a_x : Inport  Port=5
  a_y : Inport  Port=6
  Constant : Constant  Value=Q_lat_process
  Constant1 : Constant  Value=Q_lat_sensor
  Demux : Demux  Outputs=9
  MATLAB Function : MATLAB Function  TreatAsAtomicUnit=on
  MATLAB Function1 : MATLAB Function  TreatAsAtomicUnit=on
  Mux : Mux  Inputs=2
  Mux1 : Mux
  Mux2 : Mux
  Unit Delay : UnitDelay  InitialCondition=[0 V_x0 0.1 1 1 1 1 50 50]'  SampleTime=Ts
  Unit Delay1 : UnitDelay  InitialCondition=10*eye(9)  SampleTime=Ts
  r_hat : Outport
  V_x_hat : Outport  Port=2
  V_y_hat : Outport  Port=3
  F_hat_y : Outport  Port=4
  wires:
  F_zhat/1 -> Mux/2
  a_y/1 -> Mux1/4
  a_x/1 -> Mux1/3
  V_x/1 -> Mux1/2
  r/1 -> Mux1/1
  Demux/1 -> r_hat/1
  Demux/2 -> V_x_hat/1
  Demux/3 -> V_y_hat/1
  Demux/4 -> Mux2/1
  Demux/5 -> Mux2/2
  Demux/6 -> Mux2/3
  Demux/7 -> Mux2/4
  Mux2/1 -> F_hat_y/1
  delta/1 -> Mux/1
  MATLAB Function/1(X_P) -> MATLAB Function1/3(X_P)
  MATLAB Function/5(Pz_P) -> MATLAB Function1/1(Pz_P)
  MATLAB Function/4(Kk) -> MATLAB Function1/6(Kk)
  MATLAB Function/3(Z_P) -> MATLAB Function1/2(Z_P)
  MATLAB Function/2(P_P) -> MATLAB Function1/4(P_P)
  MATLAB Function1/1(X_E) -> Unit Delay/1, Demux/1
  MATLAB Function1/2(P_E) -> Unit Delay1/1
  Constant/1 -> MATLAB Function/4(Q_lat_process)
  Constant1/1 -> MATLAB Function/5(Q_lat_sensor)
  Unit Delay1/1 -> MATLAB Function/3(P_E)
  Unit Delay/1 -> MATLAB Function/1(X_E)
  Mux/1 -> MATLAB Function/2(U)
  Mux1/1 -> MATLAB Function1/5(Y)

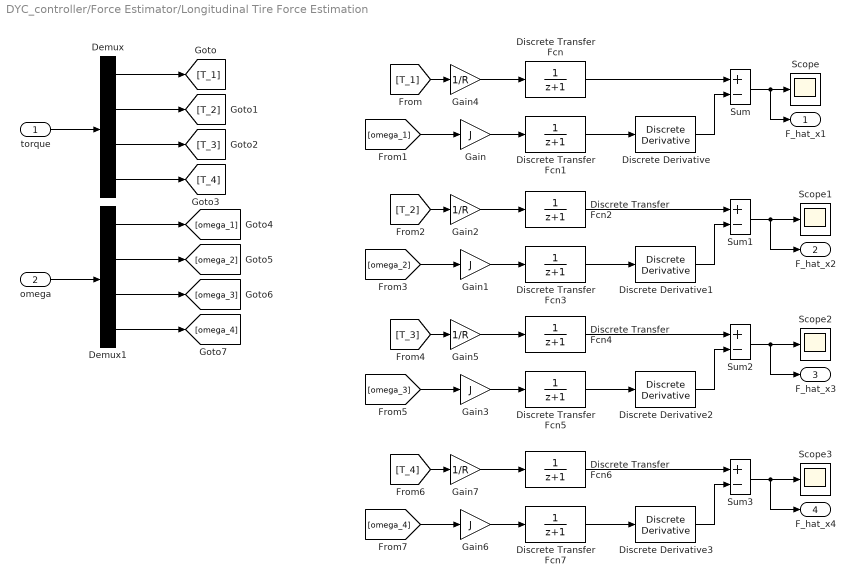
== system DYC_controller/Force Estimator/Longitudinal Tire Force Estimation ==
  torque : Inport
  omega : Inport  Port=2
  Demux : Demux
  Demux1 : Demux
  Discrete Transfer Fcn{,1..7} (8 alike) : DiscreteTransferFcn  Denominator=[1 1]  SampleTime=Ts
  Discrete Derivative{,1..3} (4 alike) : simulink/Discrete/Discrete Derivative  gainval=1.0  ICPrevScaledInput=0.0  OutMin=[]  OutMax=[]  OutDataType=fixdt(1, 16)  OutScaling=2^-10  DoSatur=off
  Gain{,1,3,6} (4 alike) : Gain  Gain=J
  Gain{2,4..5,7} (4 alike) : Gain  Gain=1/R
  Scope{,1..3} (4 alike) : Scope
  Sum{,1..3} (4 alike) : Sum  Inputs=+-
  F_hat_x1 : Outport
  F_hat_x2 : Outport  Port=2
  F_hat_x3 : Outport  Port=3
  F_hat_x4 : Outport  Port=4
  wires:
  torque/1 -> Demux/1
  omega/1 -> Demux1/1
  Demux/1 -> [T_1]
  Demux/2 -> [T_2]
  Demux/3 -> [T_3]
  Demux/4 -> [T_4]
  Demux1/1 -> [omega_1]
  Demux1/2 -> [omega_2]
  Demux1/3 -> [omega_3]
  Demux1/4 -> [omega_4]
  [T_1] -> Gain4/1
  [omega_1] -> Gain/1
  Sum/1 -> F_hat_x1/1, Scope/1
  Gain4/1 -> Discrete Transfer Fcn/1
  Gain/1 -> Discrete Transfer Fcn1/1
  Discrete Transfer Fcn/1 -> Sum/1
  Discrete Transfer Fcn1/1 -> Discrete Derivative/1
  Discrete Derivative/1 -> Sum/2
  Discrete Derivative1/1 -> Sum1/2
  Discrete Transfer Fcn3/1 -> Discrete Derivative1/1
  Discrete Transfer Fcn2/1 -> Sum1/1
  Gain1/1 -> Discrete Transfer Fcn3/1
  Gain2/1 -> Discrete Transfer Fcn2/1
  Sum1/1 -> F_hat_x2/1, Scope1/1
  [omega_2] -> Gain1/1
  [T_2] -> Gain2/1
  [T_3] -> Gain5/1
  [omega_3] -> Gain3/1
  Sum2/1 -> F_hat_x3/1, Scope2/1
  Gain5/1 -> Discrete Transfer Fcn4/1
  Gain3/1 -> Discrete Transfer Fcn5/1
  Discrete Transfer Fcn4/1 -> Sum2/1
  Discrete Transfer Fcn5/1 -> Discrete Derivative2/1
  Discrete Derivative2/1 -> Sum2/2
  Discrete Derivative3/1 -> Sum3/2
  Discrete Transfer Fcn7/1 -> Discrete Derivative3/1
  Discrete Transfer Fcn6/1 -> Sum3/1
  Gain6/1 -> Discrete Transfer Fcn7/1
  Gain7/1 -> Discrete Transfer Fcn6/1
  Sum3/1 -> Scope3/1, F_hat_x4/1
  [omega_4] -> Gain6/1
  [T_4] -> Gain7/1

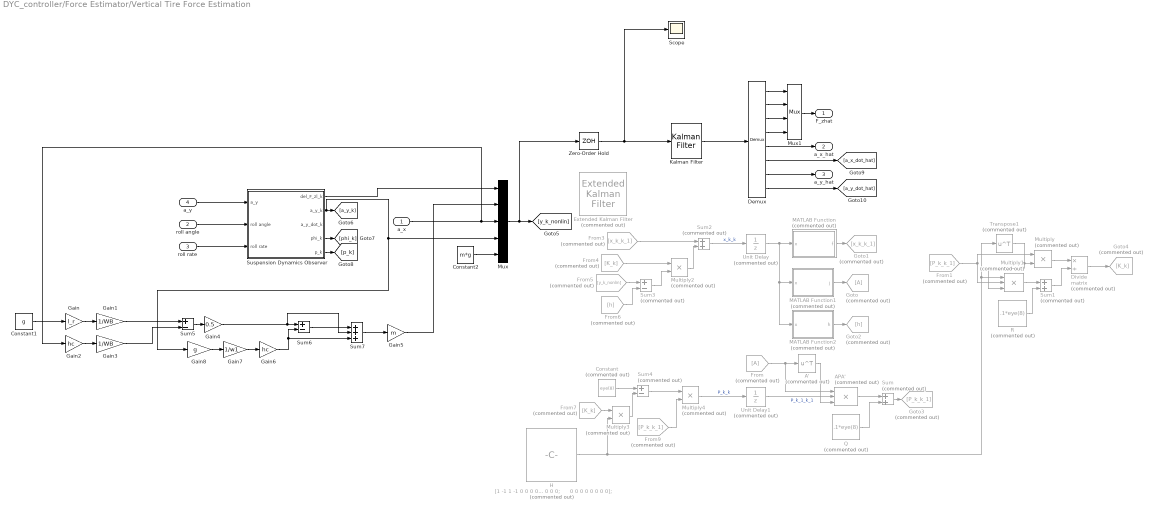
== system DYC_controller/Force Estimator/Vertical Tire Force Estimation ==
  a_x : Inport
  roll angle : Inport  Port=2
  roll rate : Inport  Port=3
  a_y : Inport  Port=4
  A' : Math  Commented=on  Operator=transpose  OutputSignalType=real  SaturateOnIntegerOverflow=on
  APA' : Product  Commented=on  Inputs=3
  Constant : Constant  Commented=on  Value=eye(8)
  Constant1 : Constant  Value=g
  Constant2 : Constant  Value=m*g
  Demux : Demux  Outputs=8
  Divide : Product  Commented=on  Inputs=*/  Multiplication=Matrix(*)
  Extended Kalman Filter : sharedTrackingLibrary/Extended Kalman Filter  Commented=on  StateTransitionFcn=vertical_force_nonlin_model  HasStateTransitionJacobianFcn=on  StateTransitionJacobianFcn=vertical_force_jacobian  HasAdditiveProcessNoise=Additive  ProcessNoise=.1*ones(8)  HasTimeVaryingProcessNoise=off  HasStateTransitionFcnExtraArgument=0  InitialState=[F_z1_s; F_z2_s; F_z3_s; F_z4_s; 0; 0; 0; 0]  InitialStateCovariance=1*ones(8)  MeasurementFcn1=vertical_force_nonlin_measurement_model  HasMeasurementJacobianFcn1=on  MeasurementJacobianFcn1=vertical_force_nonlin_measurement_jacobian  HasMeasurementEnablePort1=off  HasAdditiveMeasurementNoise1=Additive  MeasurementNoise1=.1*ones(5)  HasTimeVaryingMeasurementNoise1=off  HasMeasurementFcnExtraArgument1=0  MeasurementFcn2=myMeasurementFcn  HasMeasurementJacobianFcn2=off  HasMeasurementEnablePort2=off  HasAdditiveMeasurementNoise2=Additive  MeasurementNoise2=1  HasTimeVaryingMeasurementNoise2=off  HasMeasurementFcnExtraArgument2=0  MeasurementFcn3=myMeasurementFcn  HasMeasurementJacobianFcn3=off  HasMeasurementEnablePort3=off  HasAdditiveMeasurementNoise3=Additive  MeasurementNoise3=1  HasTimeVaryingMeasurementNoise3=off  HasMeasurementFcnExtraArgument3=0  MeasurementFcn4=myMeasurementFcn  HasMeasurementJacobianFcn4=off  HasMeasurementEnablePort4=off  HasAdditiveMeasurementNoise4=Additive  MeasurementNoise4=1  HasTimeVaryingMeasurementNoise4=off  HasMeasurementFcnExtraArgument4=0  MeasurementFcn5=myMeasurementFcn  HasMeasurementJacobianFcn5=off  HasMeasurementEnablePort5=off  HasAdditiveMeasurementNoise5=Additive  MeasurementNoise5=1  HasTimeVaryingMeasurementNoise5=off  HasMeasurementFcnExtraArgument5=0  EnableMultirate=off  StateTransitionFcnSampleTime=1  MeasurementFcn1SampleTime=1  MeasurementFcn2SampleTime=1  MeasurementFcn3SampleTime=1  MeasurementFcn4SampleTime=1  MeasurementFcn5SampleTime=1  UseCurrentEstimator=on  OutputStateCovariance=off  DataType=double  SampleTime=t_e  NumberOfMeasurements=1
      settings: SourceProductName=Control System Toolbox  SourceProductBaseCode=CT
  From : From  Commented=on
  From1 : From  Commented=on  GotoTag=P_k_k_1
  From3 : From  Commented=on  GotoTag=x_k_k_1
  From4 : From  Commented=on  GotoTag=K_k
  From5 : From  Commented=on  GotoTag=y_k_nonlin
  From6 : From  Commented=on  GotoTag=h
  From7 : From  Commented=on  GotoTag=K_k
  From9 : From  Commented=on  GotoTag=P_k_k_1
  Gain : Gain  Gain=l_r
  Gain1 : Gain  Gain=1/WB
  Gain2 : Gain  Gain=hc
  Gain3 : Gain  Gain=1/WB
  Gain4 : Gain  Gain=0.5
  Gain5 : Gain  Gain=m
  Gain6 : Gain  Gain=hc
  Gain7 : Gain  Gain=1/w1
  Gain8 : Gain  Gain=g
  Goto : Goto  Commented=on
  Goto1 : Goto  Commented=on  GotoTag=x_k_k_1
  Goto2 : Goto  Commented=on  GotoTag=h
  Goto3 : Goto  Commented=on  GotoTag=P_k_k_1
  Goto4 : Goto  Commented=on  GotoTag=K_k
  H : Constant  Commented=on  Value=|
      | [1 -1 1 -1 0 0 0 0;
      |      1 1 0 0 0 0 0 0;
      |      0 0 0 0 1 0 0 0;
      |      0 0 0 0 0 0 1 0;
      |      1 1 1 1 0 0 0 0;
      |      0 0 0 0 0 0 0 0;
      |      0 0 0 0 0 0 0 0;
      |      0 0 0 0 0 0 0 0];
  Kalman Filter : ctrlSharedLib/Kalman Filter  TimeDomain=Discrete-Time  UseCurrentEstimator=on  ModelSource=Individual A, B, C, D matrices  ModelSourceVariable=ss(0.95,1,1,0,1)  A=A_vte_p2  B=1  C=C_vte_p2  D=0  NumberOfStates=1  NumberOfInputs=1  NumberOfOutputs=1  InitialEstimateSource=Dialog  X0=[F_z1_s; F_z2_s; F_z3_s; F_z4_s; 0; 0; 0; 0]  P0=10  UseK=off  UseGH=off  NumberOfProcessNoiseInputs=1  G=1  TimeInvariantG=on  H=0  TimeInvariantH=on  Q=Q_proc_susp_p2  TimeInvariantQ=on  R=Q_meas_susp_p2  TimeInvariantR=on  N=0  TimeInvariantN=on  AddInputPort=off  AddEnablePort=off  OutputEstimatedY=off  OutputP=off  Ts=Ts
      settings: SourceProductBaseCode=CT
  MATLAB Function : MATLAB Function  Commented=on  TreatAsAtomicUnit=on
  MATLAB Function1 : MATLAB Function  Commented=on  TreatAsAtomicUnit=on
  MATLAB Function2 : MATLAB Function  Commented=on  TreatAsAtomicUnit=on
  Multiply{,2..4} (4 alike) : Product  Commented=on
  Multiply1 : Product  Commented=on  Inputs=3
  Mux : Mux  Inputs=5
  Mux1 : Mux
  Q : Constant  Commented=on  Value=.1*eye(8)
  R : Constant  Commented=on  Value=.1*eye(8)
  Scope : Scope
  Sum : Sum  Commented=on
  Sum1 : Sum  Commented=on
  Sum2 : Sum  Commented=on
  Sum3 : Sum  Commented=on  Inputs=+-
  Sum4 : Sum  Commented=on  Inputs=+-
  Sum5 : Sum  Inputs=+-
  Sum6 : Sum  Inputs=+-
  Sum7 : Sum  Inputs=+++
  Suspension Dynamics Observer : Subsystem
  Transpose1 : Math  Commented=on  Operator=transpose  SaturateOnIntegerOverflow=on
  Unit Delay : UnitDelay  Commented=on  InitialCondition=[F_z1_s; F_z2_s; F_z3_s; F_z4_s; 0; 0; 0; 0]  SampleTime=-1
  Unit Delay1 : UnitDelay  Commented=on  InitialCondition=ones(8)  SampleTime=-1
  Zero-Order Hold : ZeroOrderHold  SampleTime=Ts
  F_zhat : Outport
  a_x_hat : Outport  Port=2
  a_y_hat : Outport  Port=3
  wires:
  Unit Delay/1 -> MATLAB Function/1(x), MATLAB Function2/1(x), MATLAB Function1/1(x)
  MATLAB Function1/1(j) -> Goto/1
  MATLAB Function/1(f) -> Goto1/1
  MATLAB Function2/1(h) -> Goto2/1
  From/1 -> A'/1, APA'/1
  Unit Delay1/1 -> APA'/2  "P_k_1_k_1"
  A'/1 -> APA'/3
  APA'/1 -> Sum/1
  Q/1 -> Sum/2
  Sum/1 -> Goto3/1
  From1/1 -> Multiply1/2, Multiply/1
  H/1 -> Transpose1/1, Multiply1/1, Multiply3/2
  Multiply/1 -> Divide/1
  Sum1/1 -> Divide/2
  Transpose1/1 -> Multiply/2, Multiply1/3
  Multiply1/1 -> Sum1/1
  R/1 -> Sum1/2
  Divide/1 -> Goto4/1
  From3/1 -> Sum2/1
  From4/1 -> Multiply2/1
  Sum3/1 -> Multiply2/2
  From5/1 -> Sum3/1
  From6/1 -> Sum3/2
  Multiply2/1 -> Sum2/2
  Constant/1 -> Sum4/1
  From7/1 -> Multiply3/1
  Multiply3/1 -> Sum4/2
  Sum4/1 -> Multiply4/1
  From9/1 -> Multiply4/2
  Multiply4/1 -> Unit Delay1/1  "P_k_k"
  Sum2/1 -> Unit Delay/1  "x_k_k"
  roll angle/1 -> Suspension Dynamics Observer/2(roll angle)
  roll rate/1 -> Suspension Dynamics Observer/3(roll rate)
  a_y/1 -> Suspension Dynamics Observer/1(a_y)
  Suspension Dynamics Observer/2(a_y_k) -> Mux/4, Gain8/1, [a_y_k]
  Gain/1 -> Gain1/1
  Constant1/1 -> Gain/1
  Gain1/1 -> Sum5/1
  Gain2/1 -> Gain3/1
  Gain3/1 -> Sum5/2
  Sum5/1 -> Gain4/1
  Gain4/1 -> Sum7/2, Sum6/1
  Gain7/1 -> Gain6/1
  Gain8/1 -> Gain7/1
  Gain6/1 -> Sum7/3, Sum6/2
  Sum6/1 -> Sum7/1
  Sum7/1 -> Gain5/1
  Constant2/1 -> Mux/5
  Demux/1 -> Mux1/1
  Demux/2 -> Mux1/2
  Demux/3 -> Mux1/3
  Demux/4 -> Mux1/4
  Mux1/1 -> F_zhat/1
  Suspension Dynamics Observer/1(del_F_zl_k) -> Mux/1
  Suspension Dynamics Observer/4(phi_k) -> [phi_k]
  Suspension Dynamics Observer/5(p_k) -> [p_k]
  Demux/5 -> a_x_hat/1
  Demux/6 -> [a_x_dot_hat]
  Demux/7 -> a_y_hat/1
  Demux/8 -> [a_y_dot_hat]
  Gain5/1 -> Mux/2
  a_x/1 -> Gain2/1, Mux/3
  Mux/1 -> Zero-Order Hold/1, [y_k_nonlin]
  Kalman Filter/1 -> Demux/1
  Zero-Order Hold/1 -> Kalman Filter/1, Scope/1
